simulink model "NonLinearControlTheoryHW1C"  (R2013a)
settings: Solver=ode45  StartTime=0.0  StopTime=30  RelTol=1e-3
settings Model: Creator=Samet  LastModifiedBy=Samet

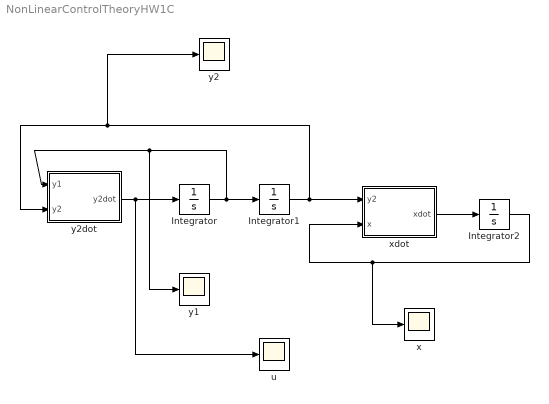
== system NonLinearControlTheoryHW1C ==
  Integrator : Integrator  InitialCondition=2.176
  Integrator1 : Integrator  InitialCondition=2.176
  Integrator2 : Integrator  InitialCondition=2.176
  u : Scope
      settings: YMin=-0.2  YMax=0.1  SaveName=ScopeData3
  x : Scope
      settings: YMin=-0  YMax=1.5  SaveName=ScopeData2
  xdot : MATLAB Function  TreatAsAtomicUnit=on
  y1 : Scope
      settings: YMin=-0.5  YMax=0
  y2 : Scope
  y2dot : MATLAB Function  TreatAsAtomicUnit=on
  wires:
  y2dot/1(y2dot) -> u/1, Integrator/1
  Integrator/1 -> y1/1, y2dot/1(y1), Integrator1/1
  Integrator1/1 -> xdot/1(y2), y2/1, y2dot/2(y2)
  xdot/1(xdot) -> Integrator2/1
  Integrator2/1 -> x/1, xdot/2(x)

== matlab function NonLinearControlTheoryHW1C/y2dot ==
  data: y1 input; y2dot output; y2 input
function y2dot = fcn(y1,y2)
alfa=10;
y2dot =-(alfa^2)*y1-2*alfa*y2;

== matlab function NonLinearControlTheoryHW1C/xdot ==
  data: y2 input; xdot output; x input
function xdot = fcn(y2,x)
xdot=-0.5*(1+y2)*x^3;
